simulink model "mcb_microchip_pmsm_foc_sensorless_dsPIC33EP256MC506"  (R2021b)
settings: Solver=FixedStepDiscrete  StartTime=0.0  StopTime=10  FixedStep=Ts  RelTol=1e-3  EnableMultiTasking=on
InitFcn:
  | mcb_microchip_pmsm_foc_sensorless_dsPIC33_data;
values from neighbouring files (symbols this model uses):
  dataType = fixdt(1,16,14)    [mcb_microchip_pmsm_foc_sensorless_dsPIC33_data.m]    (also in mcb_pmsm_foc_sensorless_dsPIC33_data.m)
  dataType2 = fixdt(1,16,12)    [mcb_microchip_pmsm_foc_sensorless_dsPIC33_data.m]    (also in mcb_pmsm_foc_sensorless_dsPIC33_data.m)
  PI_params = mcb.internal.SetControllerParameters(pmsm,inverter,PU_System,T_pwm,Ts,Ts_speed)    [mcb_microchip_pmsm_foc_sensorless_dsPIC33_data.m]    (also in mcb_pmsm_foc_sensorless_dsPIC33_data.m)
  PU_System = mcb_SetPUSystem(pmsm,inverter)    [mcb_microchip_pmsm_foc_sensorless_dsPIC33_data.m]    (also in mcb_pmsm_foc_sensorless_dsPIC33_data.m)
  PWM_frequency = 20e3    (= 20000)    [mcb_microchip_pmsm_foc_sensorless_dsPIC33_data.m]    (also in mcb_pmsm_foc_sensorless_dsPIC33_data.m)
  Speed_openLoop_PU = 0.1    [mcb_microchip_pmsm_foc_sensorless_dsPIC33_data.m]    (also in mcb_pmsm_foc_sensorless_dsPIC33_data.m)
  Ts = T_pwm    (= 5e-05)    [mcb_microchip_pmsm_foc_sensorless_dsPIC33_data.m]    (also in mcb_pmsm_foc_sensorless_dsPIC33_data.m)
  Ts_speed = 30*Ts    (= 0.0015)    [mcb_microchip_pmsm_foc_sensorless_dsPIC33_data.m]    (also in mcb_pmsm_foc_sensorless_dsPIC33_data.m)
undefined symbols (not defined in the file or in its folder): A4, C5, D8, F1, inverter, P20, P53, P97, Pin, pmsm, PWMmax
libraries: MCHP_Blockset x16, mcbcontrolslib x13, simulink x9, mcbpositiondecoderlib x2, mcbplantlib x1, autolibpmsmexterior x1
(part 1 of 3)
settings Model: Creator=M91449  LastModifiedBy=snarayan
settings SolverCC: AlgebraicLoopSolver=TrustRegion
settings DataIOCC: LimitDataPoints=on  ReturnWorkspaceOutputs=off
settings OptimizationCC: DefaultParameterBehavior=Inlined  InlineInvariantSignals=on  LifeSpan=1  EfficientTunableParamExpr=on
settings DebuggingCC: MultiTaskDSMMsg=none  SFUnexpectedBacktrackingDiag=warning  SFNoUnconditionalDefaultTransitionDiag=warning  SFExecutionAtInitializationDiag=none  SFMachineParentedDataDiag=warning  ArithmeticOperatorsInVariantConditions=warning
settings HardwareCC: ProdBitPerInt=16  ProdBitPerPointer=16  ProdBitPerSizeT=16  ProdBitPerPtrDiffT=16  ProdLargestAtomicInteger=Integer  ProdLargestAtomicFloat=None  ProdWordSize=16  ProdHWDeviceType=Generic->Custom
settings ModelReferenceCC: ModelReferenceNumInstancesAllowed=Single  PropagateSignalLabelsOutOfModel=off
settings SFSimCC: SimUseLocalCustomCode=off  MATLABDynamicMemAlloc=off  CustomCodeUndefinedFunction=UseInterfaceOnly
settings RTWCC: Description=Microchip Embedded Target PIC24 dsPIC30 dsPIC33 (real-time)  SystemTargetFile=MCHP_dsPIC_stf.tlc  TemplateMakefile=MCHP_dsPIC.tmf  GenerateReport=on  RTWUseLocalCustomCode=off  IncludeHyperlinkInReport=on  GenerateTraceInfo=on  GenerateTraceReport=on  GenerateTraceReportSl=on  GenerateTraceReportSf=on  GenerateTraceReportEml=on  GenerateCodeMetricsReport=on  GenerateCodeReplacementReport=on
settings CodeAppCC: IgnoreCustomStorageClasses=off  MaxIdLength=255  StateflowObjectComments=on
settings STFCustomTargetCC: TargetLibSuffix=_lib.a  CodeReplacementLibrary=Microchip Code Replacement Library for dsPIC  IncludeMdlTerminateFcn=off  CombineOutputUpdateFcns=on  SuppressErrorStatus=on  ERTCustomFileBanners=on  SupportContinuousTime=off  RemoveResetFunc=on  MATLABClassNameForMDSCustomization=Simulink.SoftwareTarget.ERTCustomization  GRTInterface=off  SystemTargetFile=MCHP_dsPIC_stf.tlc
settings ERTTargetCC: TargetLibSuffix=_lib.a  CodeReplacementLibrary=Microchip Code Replacement Library for dsPIC  MultiwordLength=2048  ParMdlRefBuildCompliant=off  CompOptLevelCompliant=off  ConcurrentExecutionCompliant=off  IncludeMdlTerminateFcn=off  SuppressErrorStatus=on  SupportNonInlinedSFcns=on  ModelStepFunctionPrototypeControlCompliant=off  CPPClassGenCompliant=off  UseToolchainInfoCompliant=off  InlinedParameterPlacement=NonHierarchical  ERTSrcFileBannerTemplate=MCHP_dsPIC_code_template.cgt  ERTHdrFileBannerTemplate=MCHP_dsPIC_code_template.cgt  ERTDataSrcFileTemplate=MCHP_dsPIC_code_template.cgt  ERTDataHdrFileTemplate=MCHP_dsPIC_code_template.cgt  ERTCustomFileTemplate=MCHP_main.tlc  ConvertIfToSwitch=off  SuppressUnreachableDefaultCases=off
settings ConfigComp: CovMetricSettings=dw  CovSaveCumulativeToWorkspaceVar=on  CovSaveSingleToWorkspaceVar=on  CovExternalEMLEnable=off

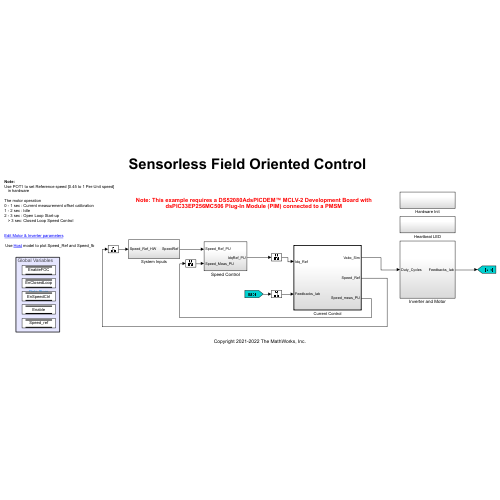
[thumbnail: Simulink's stored preview of the top-level diagram]
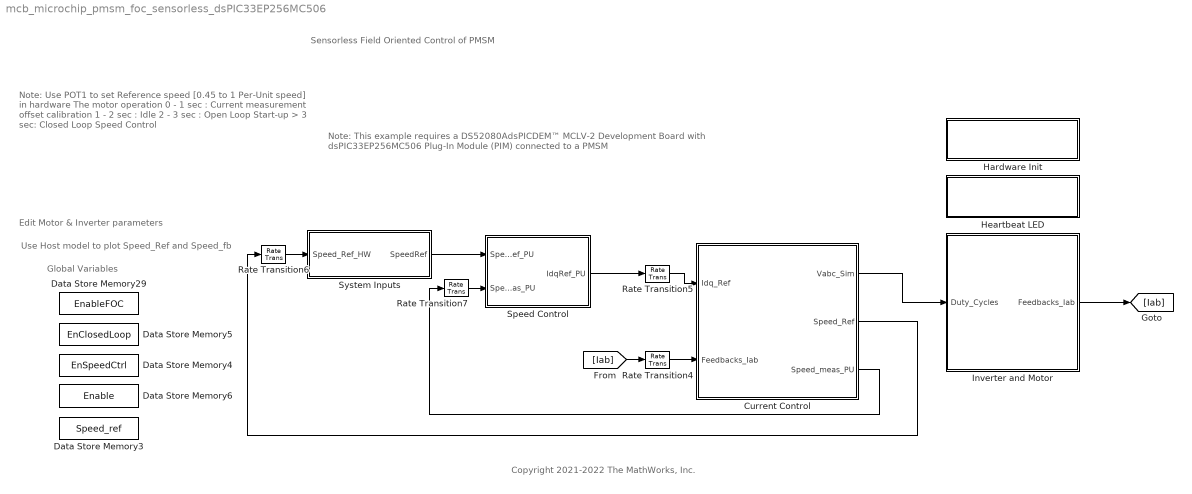
== system mcb_microchip_pmsm_foc_sensorless_dsPIC33EP256MC506 ==
  note: Use Host model to plot Speed_Ref and Speed_fb
  note: Edit Motor & Inverter parameters
  note: Note:
      | Use POT1 to set Reference speed [0.45 to 1 Per-Unit speed]
      | in hardware
      |
      | The motor operation
      | 0 - 1 sec : Current measurement offset calibration
      | 1 - 2 sec : Idle
      | 2 - 3 sec : Open Loop Start-up
      | > 3 sec: Closed Loop Speed Control
  note: Global Variables
  note: Sensorless Field Oriented Control of PMSM
  note: Note: This example requires a DS52080AdsPICDEM™ MCLV-2 Development Board with
      | dsPIC33EP256MC506 Plug-In Module (PIM) connected to a PMSM
  note: Copyright 2021-2022 The MathWorks, Inc.
  Current Control : Subsystem  TreatAsAtomicUnit=on  VariantControl=Optimized
  Data Store Memory29 : DataStoreMemory  DataStoreName=EnableFOC  ShowAdditionalParam=off  OutDataTypeStr=boolean
  Data Store Memory3 : DataStoreMemory  DataStoreName=Speed_ref  ReadBeforeWriteMsg=warning  WriteAfterWriteMsg=warning  WriteAfterReadMsg=warning  InitialValue=0.1  ShowAdditionalParam=off  OutDataTypeStr=dataType
  Data Store Memory4 : DataStoreMemory  DataStoreName=EnSpeedCtrl  ReadBeforeWriteMsg=warning  WriteAfterWriteMsg=warning  WriteAfterReadMsg=warning  ShowAdditionalParam=off  OutDataTypeStr=boolean
  Data Store Memory5 : DataStoreMemory  DataStoreName=EnClosedLoop  ReadBeforeWriteMsg=warning  WriteAfterWriteMsg=warning  WriteAfterReadMsg=warning  ShowAdditionalParam=off  OutDataTypeStr=boolean
  Data Store Memory6 : DataStoreMemory  DataStoreName=Enable  ShowAdditionalParam=off  OutDataTypeStr=boolean
  Hardware Init : Subsystem
  Heartbeat LED : Subsystem
  Inverter and Motor : Subsystem
  Rate Transition4 : RateTransition  Deterministic=off
  Rate Transition5 : RateTransition  Deterministic=off
  Rate Transition6 : RateTransition  Deterministic=off  OutPortSampleTime=Ts_speed
  Rate Transition7 : RateTransition  Deterministic=off  OutPortSampleTime=Ts_speed
  Speed Control : Subsystem  SystemSampleTime=Ts_speed
  System Inputs : Subsystem
  wires:
  Current Control/1(Vabc_Sim) -> Inverter and Motor/1(Duty_Cycles)
  Rate Transition4/1 -> Current Control/2(Feedbacks_Iab)
  Rate Transition7/1 -> Speed Control/2(Speed_Meas_PU)
  Speed Control/1(IdqRef_PU) -> Rate Transition5/1
  Current Control/3(Speed_meas_PU) -> Rate Transition7/1
  Inverter and Motor/1(Feedbacks_Iab) -> [Iab]
  [Iab] -> Rate Transition4/1
  Rate Transition5/1 -> Current Control/1(Idq_Ref)
  Current Control/2(Speed_Ref) -> Rate Transition6/1
  Rate Transition6/1 -> System Inputs/1(Speed_Ref_HW)
  System Inputs/1(SpeedRef) -> Speed Control/1(Speed_Ref_PU)

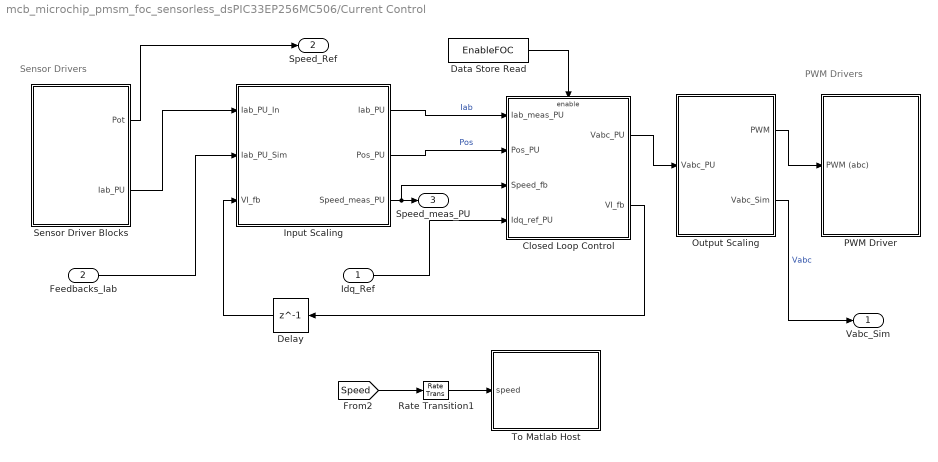
== system mcb_microchip_pmsm_foc_sensorless_dsPIC33EP256MC506/Current Control ==
  note: Sensor Drivers
  note: PWM Drivers
  Idq_Ref : Inport
  Feedbacks_Iab : Inport  Port=2
  Closed Loop Control : Subsystem
  Data Store Read : DataStoreRead  DataStoreName=EnableFOC  IndexOptions=Index vector (dialog)  Indices=1  OutputSizes=1
  Delay : Delay  DelayLength=1
  Input Scaling : Subsystem
  Output Scaling : Subsystem
  PWM Driver : Subsystem
  Rate Transition1 : RateTransition
  Sensor Driver Blocks : Subsystem
  "To Matlab Host " : Subsystem
  Vabc_Sim : Outport
  Speed_Ref : Outport  Port=2
  Speed_meas_PU : Outport  Port=3
  wires:
  Closed Loop Control/1(Vabc_PU) -> Output Scaling/1(Vabc_PU)
  Output Scaling/1(PWM) -> PWM Driver/1(PWM (abc))
  Feedbacks_Iab/1 -> Input Scaling/2(Iab_PU_Sim)
  Input Scaling/1(Iab_PU) -> Closed Loop Control/1(Iab_meas_PU)  "Iab"
  Input Scaling/2(Pos_PU) -> Closed Loop Control/2(Pos_PU)  "Pos"
  Sensor Driver Blocks/1(Pot) -> Speed_Ref/1
  Sensor Driver Blocks/2(Iab_PU) -> Input Scaling/1(Iab_PU_In)
  Rate Transition1/1 -> "To Matlab Host "/1(speed)
  [Speed] -> Rate Transition1/1
  Closed Loop Control/2(VI_fb) -> Delay/1
  Delay/1 -> Input Scaling/3(VI_fb)
  Idq_Ref/1 -> Closed Loop Control/4(Idq_ref_PU)
  Output Scaling/2(Vabc_Sim) -> Vabc_Sim/1  "Vabc"
  Input Scaling/3(Speed_meas_PU) -> Closed Loop Control/3(Speed_fb), Speed_meas_PU/1
  Data Store Read/1 -> Closed Loop Control/Enable

== system mcb_microchip_pmsm_foc_sensorless_dsPIC33EP256MC506/Hardware Init ==
  Compiler Options : MCHP_Blockset/System Configuration/Compiler Options  Priority=1  LATEST_CMPLR=on  COMP_LIST=Dynamic Options  COMP_LIST_TXT=xc16 - v1.70  DFP_LIST=Dynamic Options  DFP_LIST_TXT=Dynamic Options  CMSIS_DSP=Dynamic Options  CMSIS_DSP_TXT=Dynamic Options  USE_64BIT_DOUBLE=off  MCHP_MULTITHREAD_COMPILATION=on  UseCustom_LinkerScript=off  MCHP_MASTERLINK=mcb_pmsm_foc_sensorless_dsPIC33EP256MC506/Hardware Init/Microchip Master  OPTIMIZATION_LEVEL=3  OPTIMIZATION_FLTO=on  OPTIMIZATION_REORDER=off  UNROLL_LOOPS=on  PROCEDURAL_ABSTRACTION=off  MPLAB_LINKLIB=default  MPLAB_LINKLIB1=default  MCODE=is less than 32768 (faster)  MCONST=in data memory  MDATA=Use only memory below address 8192 (faster)  MSCALAR=Use only memory below address 8192 (faster)  MLARGEARRAY=off  MAGGREGATE=off  HEAP_SIZE=0  OMF=elf  DEBUG_INFO=off  ProduceHexOutput=on  AssemblyListing=off  NO_EDS_WARN=on  PRINT_STATISTICS=off
      settings: SourceProductName=MPLAB Device Blocks for Simulink
  Data Sheet : MCHP_Blockset/System Info/Data Sheet  DOC_Type=datasheet  DOC_MCHP_Id=33EP256MC506_datasheet  DOC_FilePath=C:\Users\M91449\AppData\Local\Temp\70000657H.pdf  DOC_FileLastCheckTime="[2016              1             28             13             25         44.133]"  cpy_MCHP_Id=33EP256MC506  MCHP_MASTERLINK=mcb_pmsm_foc_sensorless_dsPIC33EP256MC506/Hardware Init/Microchip Master
      settings: AttributesFormatString=%<cpy_MCHP_Id>  SourceProductName=MPLAB Device Blocks for Simulink
  Microchip Master : MCHP_Blockset/System Configuration/Microchip Master  Priority=1  PICREF=33EP256MC506  TIMESTEP_REF=ADC  BUSYFLAG=Dynamic Options  BUSYFLAG_TXT=D8 / Pin[42]  PWRTEN=Not used  BOREN=Disable  BODENV=2.7V  BORV=Not used  FPWRT=128ms  DSBOREN=Enable ZPBOR during Deep Sleep Mode  DSLPBOR=Not used  MCLRE=Enabled  SMCLR=MCLR pin generates a normal system Reset  PMDL1WAY=Allow only one reconfiguration  RSTPRI=Device will obtain reset instruction from Primary flash  TEMP=Not used  SOSCSRC=Not used  SOSCSEL=Not used  IOL1WAY=Allow only one reconfiguration  ALTVREF=Not used  DISUVREG=Not used  DSSWEN=Not used  LPCFG=Not used  RTCBAT=Not used  VBTBOR=Not used  WUTSEL=Not used  POWERSAVE=off  FNOSC=Primary Oscillator (XT; HS; EC)  FPR=ECIO w/ PLL 16x  FOSFPR=HS3 w/PLL 16x  FOS=Primary Oscillator  FRANGE=High Range  OSCILLATOR_SELECT=Crystal / Ceramic resonator  OSCILLATOR_SELECT_spd=Crystal / Ceramic resonator  QUARTZ=8e6  QUARTZ_spd=8e6  POSCGAIN=2x gain setting  POSCBOOST=Boost the kick start of the oscillator  SOSCGAIN=2x gain setting  SOSCBOOST=Boost the kick start of the oscillator  ACTIV_PLL=on  ACTIV_PLL_spd=on  MIPS_DESIRED=70e6  MIPS_DESIRED_spd=70e6  FPLLMUL=Not used  FPLLIDIV=8x Divider  POSCFREQ=Not used  POSCMD=XT Crystal Oscillator Mode  POSCMOD=Primary Oscillator Disabled  MIPS=70 * 1e6  ACLKCON=Optimized for PWM resolution & ADC conversion speed  ACLKCON_spd=Optimized for PWM resolution & ADC conversion speed  FPLLODIV=32x Divider  PLLKEN=Clock switch to PLL source will wait until the PLL lock signal is valid.  FCKSM=Both Clock switching and Fail-safe Clock Monitor are enabled  FCKSMEN=Sw Disabled; Mon Disabled  IESO=Start up with FRC; then switch  DSWDTPS=1:2^36  FWDTEN=Disable  FWDTWINSZ=Window size is 25%  FWPSA=1:512  FWPSA0=1:128  FWPSB=1:16  WDT=Disable  WDTPOST=1:32768  WDTPRE=1:128  WDTPS=1:32768  WINDIS=Watchdog Timer in Non-Window mode  WWDTEN=Non-Window mode  DSWDTEN=Enable DSWDT during Deep Sleep Mode  DSWDTOSC=Select LPRC as DSWDT Reference clock  FPBDIV=Not used  FSOSCEN=Disable Secondary Oscillator  LPRCSEL=Not used  OSCIOFCN=Not used  OSCIOFNC=general purpose digital I/O pin  LVRCFG=Not used  PLL_96MHZ=Not used  PLL96MHZ=Not used  PLLDIV=Not used  WDTCLK=Not used  WDTCMX=Not used  WDTWIN=WDT Window is 25% of WDT period  XTCFG=24-32 MHz crystals  XTBST=Boost the kick-start  APL=Aux Flash Code protect is disabled  APLK=Aux Flash Write Protection or Code Protection is Enabled  AWRP=Auxiliary program memory is not write-protected  BSS=No Boot program Flash segment  BWP=Not used  BWRP=Boot Segment may be written  CP=Protection Disabled  EBS=No Boot EEPROM  ESS=No Segment Data EEPROM  GCP=General Segment Code protect is Disabled  GSS=General Segment Code protect is Disabled  GSS0=Not used  GSSK=General Segment Write Protection or Code Protection is Enabled  GWRP=General Segment may be written  PWP=Not used  RBS=No Boot RAM  RSS=No Secure RAM  SSS=No Secure Segment  SWRP=Secure segment may be written  WPCFG=Not used  WPDIS=Not used  WPEND=Not used  WPFP=Not used  ICESEL=Communicate on PGEC1/PGED1  ICS=Communicate on PGEC2 and PGED2  JTAGEN=Disable  COE=Not used  RES=Not used  DEBUG=Debugger is disabled  BACKBUG=Not used  BKBUG=Not used  ALTI2C=I2C mapped to SDA1/SCL1 pins  ALTI2C1=I2C1 mapped to SDA1/SCL1 pins  ALTI2C2=I2C2 mapped to SDA2/SCL2 pins  ALTI2C3=I2C3 mapped to SDA3/SCL3 pins  ALTQIO=QEA1; QEB1; INDX1 are selected as inputs to QEI1  ALTSS1=SS1A is selected as the I/O pin for SPI1  CMPPOL0=Hysteresis is applied to falling edge  CMPPOL1=Hysteresis is applied to falling edge  FCANIO=Not used  FETHIO=Default Ethernet I/O  FMIIEN=MII Enabled  FSRSSEL=Not used  FUSBIDIO=Controlled by the USB Module  FVBUSONIO=Not used  HPOL=PWM module high side output pins have active-high output polarity  HYST0=45 mV Hysteresis  HYST1=45 mV Hysteresis  I2C1SEL=Not used  LPOL=PWM module low side output pins have active-high output polarity  PWMPIN=PWM module pins controlled by PORT register at device Reset  RTCOSC=Not used  UPLLEN=USB PLL Disabled  UPLLIDIV=Not used  ATMOD8=Not used  ALTPMP=Not used  I2C2SEL=Not used  ALTADREF=Not used  ALTCVREF=Not used  PWMLOCK=PWM registers may be written without key sequence  INT_PRIORITY_DMA=0  MCHP_TIMER_RESULT=[ ]  MCHP_PORT={Busy Flag}{Busy}0:1:D8;  MCHP_PLLRegisters="[5    243  16385     -1     -1]"  MCHPVAR=MCHP.fcy.MIPS=70000000;MCHP.fcy.SYSCLK=70000000;MCHP.fcy.ADC=70000000;MCHP.fcy.Comparator=70000000;MCHP.fcy.I2C=70000000;MCHP.fcy.SPI=70000000;MCHP.fcy.UART=70000000;MCHP.fcy.Timers=70000000;MCHP.fcy.OC=70000000;MCHP.fcy.IC=70000000;MCHP.fcy.Ports=70000000;MCHP.fcy.QEI=70000000;MCHP.PowerSave=0;MCHP.TimeStepFactor=-1000;MCHP.TimeStep_Timer=-1;MCHP.NTIMERS=5;MCHP.id.name='33EP256MC506';MCHP.id.N=reshape([33 256 506],1,3);MCHP.id.L=reshape({ 'EP','MC',''},1,3);MCHP.id.Arch=3;MCHP.periph.PPS.reg_RPINRx=reshape([-1 1 1 -1 -1 -1 1 -1 -1 -1 -1 -1 -1 -1 1 1 1 1 -1 -1 -1 -1 -1 -1 1 1 -1 -1 1 1 1 1 -1 -1 -1 -1 1 -1 1 -1 -1 -1 -1 -1 1 1 1 -1 -1 -1 -1 -1 1 -1 -1 -1 -1 -1 -1 -1 -1 -1 -1 -1 -1 -1 -1 -1 -1 -1 -1 -1 -1 -1 -1 1 -1 1 1 1],1,80);MCHP.PPS.dsPIC.RP=reshape([-1 -1 -1 -1 -1 -1 -1 -1 -1 -1 -1 -1 -1 -1 -1 -1 -1 -1 -1 -1 4 -1 -1 -1 -1 -1 -1 -1 -1 -1 -1 -1 -1 -1 -1 19 20 21 22 23 24 25 26 27 -1 -1 -1 -1 -1 -1 -1 -1 -1 -1 38 39 40 41 -1 -1 -1 -1 -1 -1 -1 -1 -1 -1 -1 -1 -1 -1 -1 -1 -1 -1 -1 -1 -1 -1 -1 -1 -1 -1 -1 -1 -1 -1 -1 -1 -1 -1 -1 -1 -1 -1 -1 81 -1 -1 -1 -1 -1 -1 -1 -1 -1 -1 -1 -1 -1 -1 -1 -1 -1 -1 -1 -1 102 -1 104],1,121);MCHP.PPS.dsPIC.RPI=reshape([-1 -1 -1 -1 -1 -1 -1 -1 -1 -1 -1 -1 -1 -1 -1 -1 -1 -1 -1 -1 -1 -1 -1 -1 8 9 -1 11 12 -1 -1 -1 16 17 18 -1 -1 -1 -1 -1 -1 -1 -1 -1 28 29 30 31 -1 -1 -1 35 36 37 -1 -1 -1 -1 42 -1 -1 -1 -1 -1 -1 -1 -1 -1 -1 -1 -1 -1 -1 -1 -1 -1 -1 -1 -1 -1 -1 -1 -1 -1 -1 -1 -1 -1 -1 -1 -1 -1 -1 -1 78 79 80 -1 -1 -1 -1 -1 -1 -1 -1 -1 -1 -1 -1 -1 -1 -1 -1 -1 -1 -1 -1 -1 -1 103 -1 105],1,122);MCHP.PPS.dsPIC.RPINR_list=reshape({ '1','INT1','INT2','INT3','INT4','T1CK','T2CK','T3CK','T4CK','T5CK','T6CK','T7CK','T8CK','T9CK','IC1','IC2','IC3','IC4','IC5','IC6','IC7','IC8','OCFA','OCFB','FLT1','FLT2','FLT3','FLT4','QEIA1','QEIB1','QEINDX1','QEIHOM1','QEIA2','QEIB2','QEINDX2','QEIHOM2','U1RX','U1CTS','U2RX','U2CTS','SDI1','SCK1_in','SS1_in','44','SDI2','SCK2_in','SS2_in','48','CSDIR','CSCK','COFS','52','C1RX','C2RX','U3RX','U3CTS','U4RX','U4CTS','SDI3','SCK3_in','SS3_in','62','SDI4','SCK4_in','SS4_in','66','IC9','IC10','IC11','IC12','IC13','IC14','IC15','IC16','OCFC','SYNCI1','SYNCI2','DTCMP1','DTCMP2','DTCMP3','DTCMP4','DTCMP5','DTCMP6','DTCMP7','FLT5','FLT6','FLT7','FLT8','89','SENT1','SENT2','92'},1,92);MCHP.PPS.dsPIC.RPOR_list=reshape({ '1','U1TX','U1RTS','U2TX','U2RTS','SDO1','SCK1_out','SS1_out','SDO2','SCK2_out','SS2_out','CSDO','CSCK','COFS','C1TX','C2TX','OC1','OC2','OC3','OC4','OC5','OC6','OC7','OC8','C1OUT','C2OUT','C3OUT','U3TX','U3RTS','U4TX','U4RTS','SDO3','SCK3_out','SS3_out','SDO4','SCK4_out','SS4_out','OC9','OC10','OC11','OC12','OC13','OC14','OC15','OC16','SYNCO1','SYNCO2','QEI1CCMP','QEI2CCMP','REFCLK','C4OUT','C5OUT','52','53','54','55','56','SENT1','SENT2'},1,59);MCHP.PPS.map_RPnR_RPORx=reshape([20 35 36 37 38 39 40 41 42 43 54 55 56 57 -1 97 -1 118 120],1,19);MCHP.Rx=reshape([13 15 21 -1 -1 58 -1 -1 -1 -1 -1 14 16 22 -1 -1 59 -1 -1 -1 -1 -1 -1 17 23 -1 -1 -1 -1 -1 -1 -1 -1 -1 18 35 -1 -1 -1 -1 -1 -1 -1 -1 33 32 36 -1 -1 -1 -1 -1 -1 -1 -1 -1 43 37 53 -1 -1 -1 -1 -1 -1 -1 -1 44 50 54 -1 -1 4 -1 -1 -1 -1 1 46 51 -1 -1 -1 5 -1 -1 -1 -1 31 48 52 42 -1 -1 6 -1 -1 -1 -1 34 49 55 -1 -1 -1 8 -1 -1 -1 -1 64 60 45 -1 -1 -1 -1 -1 -1 -1 -1 12 61 24 -1 -1 -1 -1 -1 -1 -1 -1 11 62 39 -1 27 -1 -1 -1 -1 -1 -1 -1 63 47 -1 28 -1 -1 -1 -1 -1 -1 -1 2 -1 -1 29 -1 -1 -1 -1 -1 -1 -1 3 40 -1 30 -1 -1 -1 -1 -1 -1],11,16);MCHP.ADC.ANtype=reshape([3 0],1,2);MCHP.ADC.ADCONx=reshape([47103 59391 40959 263 0 0],1,6);MCHP.ADC.ADCHS_0=reshape([40863 1799],1,2);MCHP.ADC.Flags=reshape([1 0],1,2);MCHP.ADC.Buffer=reshape([16 -1],1,2);MCHP.ADC.port=reshape([0 1 16 17 18 19 32 33 34 11 12 43 76 77 78 79 -1 -1 -1 -1 -1 -1 -1 -1 -1 -1 -1 -1 -1 -1 -1 -1 -1 -1 -1 -1 -1 -1 -1 -1 -1 -1 -1 -1 -1 -1 -1 -1 -1 -1 -1 -1 -1 -1 -1 -1 -1],1,57);MCHP.ADC.port_ALT=reshape([-1 -1 -1 -1],1,4);MCHP.ADC.port_VrefP=17;MCHP.ADC.port_VrefM=16;MCHP.ADC.port_AVdd=-1;MCHP.ADC.port_AVss=-1;MCHP.ADC.ADCDATA=reshape([0 0 0 0 0 0 0 0 0 0 0 0 0 0 0 0 0 0 0 0 0 0 0 0 0 0 0 0 0 0 0 0 0 0 0 0 0 0 0 0 0 0 0 0 0 0 0 0 0 0 0 0 0 0 0 0 0],1,57);MCHP.ADC.HS_SAR.TRGSRC=reshape([0 0 0 0 0 0 0 0 0 0 0 0 0 0 0 0 0 0 0 0 0 0 0 0 0 0],1,26);MCHP.ADC.HS_SAR.nFilters=0;MCHP.ADC.HS_SAR.nDedicatedCore=0;MCHP.ADC.HS_SAR.CALIBRATION=0;MCHP.ADC.HS_SAR.ADCON1L=-1;MCHP.ADC.HS_SAR.ADC_Class3_idxStart=32;MCHP.memory.RAM=32768;MCHP.memory.RAM_XBegin=4096;MCHP.memory.RAM_YBegin=20480;MCHP.memory.RAM_dma=reshape([-1 -1],1,2);MCHP.memory.FLASH_ECC=0;MCHP.DMA.Num=4;MCHP.DMA.CNTmax=16383;MCHP.QEI.QEICONx=reshape([49023 -1 -1 -1 -1 -1],1,6);MCHP.QEI.QEItype=1;MCHP.QEI.Port_QEI_INDX=reshape([-1 -1],1,2);MCHP.QEI.Port_QEI_QEA=reshape([-1 -1],1,2);MCHP.QEI.Port_QEI_QEB=reshape([-1 -1],1,2);MCHP.QEI.Port_QEI_UPDN=reshape([-1 -1],1,2);MCHP.INT.Port=reshape([23 32767 32767 -1 -1],1,5);MCHP.PWM_HS.Flags=reshape([3 1 0],1,3);MCHP.PWM.port_FLT=reshape([-1 -1 -1 34 43 -1 -1 -1 -1 -1 -1 -1 -1 -1 -1 -1 -1 -1 -1 -1 -1 -1 -1 -1 -1 -1 -1 -1 -1 -1 -1 -1 20],1,33);MCHP.PWM.PWMRef=-1;MCHP.PWM.Flag=0;MCHP.PWM.Port_PWM_l=reshape([31 -1 29 -1 27 -1 -1 -1 -1 -1 -1 -1 -1 -1 -1 -1 -1 -1 -1 -1 -1 -1 -1 -1],2,12);MCHP.PWM.Port_PWM_h=reshape([30 -1 28 -1 26 -1 -1 -1 -1 -1 -1 -1 -1 -1 -1 -1 -1 -1 -1 -1 -1 -1 -1 -1],2,12);MCHP.PWM_HS_FEP.nEVTOUT=-1;MCHP.IC.Port=reshape([32767 32767 32767 32767 0 0 0 0 0 0 0 0 0 0 0 0],1,16);MCHP.IC.type=1;MCHP.OC.Port=reshape([32767 32767 32767 32767 0 0 0 0 0 0 0 0 0 0 0 0],1,16);MCHP.OC.type=1;MCHP.CN.Port=reshape([-1 -1 -1 -1 -1 -1 -1 -1 -1 -1 -1 -1 -1 -1 -1 -1 -1 -1 -1 -1 -1 -1 -1 -1 -1 -1 -1 -1 -1 -1 -1 -1 -1 -1 -1 -1 -1 -1 -1 -1 -1 -1 -1 -1 -1 -1 -1 -1 -1 -1 -1 -1 -1 -1 -1 -1 -1 -1 -1 -1 -1 -1 -1 -1 -1 -1 -1 -1 -1 -1 -1 -1 -1 -1 -1 -1 -1 -1 -1 -1 -1 -1 -1 -1 -1],1,85);MCHP.CN.PullUp=reshape([8083 65535 49151 352 61440 3 960 0 0 0 0],1,11);MCHP.CN.type=1;MCHP.CN.Flag_PullDown=1;MCHP.SPI.Refs=reshape([1 2 0 0 0 0],1,6);MCHP.SPI.SPIxCON1=8191;MCHP.SPI.SPIxCON2=57347;MCHP.SPI.Port_SDI=reshape([9 -1 -1 -1 -1 -1],1,6);MCHP.SPI.Port_SDO=reshape([4 -1 -1 -1 -1 -1],1,6);MCHP.SPI.Port_SCK=reshape([35 -1 -1 -1 -1 -1],1,6);MCHP.SPI.Port_SS=reshape([16 -1 -1 -1 -1 -1],1,6);MCHP.I2C.Refs=reshape([1 2 0 0 0],1,5);MCHP.I2C.I2CxCON=49151;MCHP.I2C.NewRegName=1;MCHP.I2C.Port_SDA=reshape([36 8 -1 -1 -1],1,5);MCHP.I2C.Port_SCL=reshape([37 20 -1 -1 -1],1,5);MCHP.I2C.Port_ASDA=reshape([25 21 -1 -1 -1],1,5);MCHP.I2C.Port_ASCL=reshape([24 22 -1 -1 -1],1,5);MCHP.I2C.Fuse_Port_SCL_SDA=reshape([3 1 4 1 -1 -1 -1 -1 -1 -1],2,5);MCHP.I2C.Fuse_Port_ASCL_ASDA=reshape([3 2 4 2 -1 -1 -1 -1 -1 -1],2,5);MCHP.SCCP.nSCCP=0;MCHP.SCCP.MCCP=reshape([0 0 0 0 0 0 0 0 0],1,9);MCHP.PGA.Port_PGA1P=reshape([-1 -1 -1 -1],1,4);MCHP.PGA.Port_PGA1N=reshape([-1 -1 -1 -1],1,4);MCHP.PGA.Port_PGA2P=reshape([-1 -1 -1 -1],1,4);MCHP.PGA.Port_PGA2N=reshape([-1 -1 -1 -1],1,4);MCHP.PGA.Num=0;MCHP.HS_AnalogComparator.Port_CMP1=reshape([-1 -1 -1 -1],1,4);MCHP.HS_AnalogComparator.Port_CMP2=reshape([-1 -1 -1 -1],1,4);MCHP.HS_AnalogComparator.Port_CMP3=reshape([-1 -1 -1 -1],1,4);MCHP.HS_AnalogComparator.Port_CMP4=reshape([-1 -1 -1 -1],1,4);MCHP.HS_AnalogComparator.PORT_EXTREFx=reshape([-1 -1],1,2);MCHP.HS_AnalogComparator.Port_DACOUTx=reshape([-1 -1],1,2);MCHP.HS_AnalogComparator.Num=0;MCHP.Comp.Port_CVrefin=-1;MCHP.Comp.Port_CVref=-1;MCHP.Comp.Port_CVref1O=24;MCHP.Comp.Port_CVref2O=4;MCHP.Comp.Port_CxOUT=reshape([32767 32767 32767 32767 -1],1,5);MCHP.Comp.Port_OAxOUT=reshape([17 0 32 -1 -1],1,5);MCHP.Comp.Port_CxINP=reshape([18 1 34 32 -1],1,5);MCHP.Comp.Port_CxINM=reshape([19 43 -1 -1 16 76 -1 -1 33 77 -1 -1 33 -1 -1 -1 -1 -1 -1 -1],4,5);MCHP.Comp.Port_OAxINP=reshape([-1 -1 -1 -1 -1],1,5);MCHP.Comp.Port_OAxINM=reshape([-1 -1 -1 -1 -1],1,5);MCHP.Comp.nComp=reshape([4 0 0],1,3);MCHP.Comp.OpAmp=7;MCHP.Comp.CVRCON=reshape([17663 0],1,2);MCHP.Comp.CMCON=0;MCHP.CDAC.Port_DACx=reshape([-1 -1 -1],1,3);MCHP.CDAC.nCDAC=0;MCHP.UART.port_Rx=reshape([32767 32767 -1 -1 -1 -1],1,6);MCHP.UART.port_Tx=reshape([32767 32767 -1 -1 -1 -1],1,6);MCHP.UART.port_ARx=reshape([-1 -1],1,2);MCHP.UART.port_ATx=reshape([-1 -1],1,2);MCHP.UART.port_RTS=reshape([34 76 -1 -1 -1 -1],1,6);MCHP.UART.port_CTS=reshape([43 77 -1 -1 -1 -1],1,6);MCHP.UART.reg_UxMODE=reshape([48127 48127 -1 -1 -1 -1],1,6);MCHP.UART.reg_UxSTA=reshape([61439 61439 -1 -1 -1 -1],1,6);MCHP.modsrc.DOS_02551_cpu_16bit_v7=0;MCHP.modsrc.DOS_01520_wdt_dmt_upb_v1_16bit=0;MCHP.modsrc.DOS_02359a_sent_j2716_upb_v1=0;MCHP.modsrc.DOS_02672_math_progcrc_upb_v1_16bit=0;MCHP.modsrc.DOS_01577_cla_clc_upb_v1=0;MCHP.modsrc.DOS_02915_ecc_v2=0;MCHP.modsrc.DOS_02673_tmr_classa_upb_v1_16bit=0;MCHP.modsrc.DOS_01494_qei_32b_upb_v1_16bit=0;MCHP.modsrc.DOS_02552_msi_upb_v1_Master=0;MCHP.modsrc.DOS_01441_i2c_upb_v1_16bit_TLAH=0;MCHP.modsrc.DOS_03076_uart_protocol_upb_v1_16bit=0;MCHP.modsrc.DOS_01482=0;MCHP.modsrc.DOS_01483_pwm_16bit=0;MCHP.modsrc.DOS_02497_WACV=0;MCHP.modsrc.DOS_02316_nvm_ctrl_v1_16bit=0;MCHP.modsrc.DOS_02653_afe_current_bias_ctrl_upb_v1_16bit=0;MCHP.modsrc.DOS_01459_ptg_pc_upb_v1_16bit=0;MCHP.modsrc.DOS_01512_ccp_mccp_upb_v1_16bit=0;MCHP.modsrc.DOS_02519_dma_sfr_16bit_v2=0;MCHP.modsrc.DOS_02508c11=0;MCHP.modsrc.DOS_02475_dac_pdm_nbit_upb_v1_16bit=0;MCHP.modsrc.DOS_02467_gpio_upb_v1_16bit=0;MCHP.modsrc.DOS_00805_rst_integration_v4=0;MCHP.modsrc.DOS_02659_clk_sib_v12=0;MCHP.modsrc.DOS_02674_wdt_upb_v1_16bit=0;MCHP.modsrc.DOS_01407=0;MCHP.modsrc.DOS_02552_msi_upb_v1_Slave=0;MCHP.modsrc.DOS_02593_amp_pga_ctrl_pb_v2_16bit=0;MCHP.modsrc.DOS_03247_CAN_FD_UPB_V2_16_bit=0;MCHP.modsrc.DOS_01461_afe_ctmu_con_upb_v1_16bit=0;MCHP.modsrc.DOS_02497_WACA=0;MCHP.modsrc.DOS_02478_uart_irda_upb_v1_16bit=0;MCHP.modsrc.DOS_00929=1;MCHP.modsrc.DOS_01198=1;MCHP.modsrc.DOS_03029_WACH=0;MCHP.modsrc.DOS_02949_WACG=0;MCHP.modsrc.DOS_03349_amp_pad_opamp_ctrl_upb_v1=0;MCHP.modsrc.DOS_02237_osc_dco_ctrl_upb_v1_16bit=0;MCHP.modsrc.DOS_02472_ppi_pmp16_upb_v1_16bit=0;MCHP.modsrc.DOS_03994_WAC07=0;MCHP.modsrc.DOS_03662_WACU=0;MCHP.modsrc.DOS_00794=1;MCHP.modsrc.DOS_00931=1;MCHP.modsrc.DOS_00932=1;MCHP.modsrc.DOS_00942=1;MCHP.modsrc.DOS_00938=1;MCHP.modsrc.DOS_00996=1;MCHP.modsrc.DOS_00997=1;MCHP.modsrc.DOS_00998=1;MCHP.modsrc.DOS_00209=0;MCHP.modsrc.DOS_01555_adc=0;MCHP.modsrc.DOS_01293=1;MCHP.modsrc.DOS_00828=0;MCHP.modsrc.DOS_01116=1;MCHP.modsrc.DOS_01017_RPORx=1;MCHP.modsrc.DOS_01017_RPINRx=1;MCHP.modsrc.DOS_01555_nvm_tsmc18_v2_16bit=0;MCHP.modsrc.DOS_00804=1;MCHP.modsrc.DOS_00826=1;MCHP.modsrc.DOS_01555_TLAK_PMDx=0;MCHP.modsrc.DOS_01555_TLAK_INT_=0;MCHP.modsrc.DOS_00933=1;MCHP.modsrc.DOS_01555=0;MCHP.modsrc.DOS_01555_ptg=0;MCHP.modsrc.DOS_00958=1;MCHP.modsrc.DOS_01117_PORTx=1;MCHP.modsrc.DOS_00999=0;MCHP.modsrc.DOS_01041=1;MCHP.modsrc.DOS_00892=1;MCHP.modsrc.DOS_01287_TLAC_PMDx=1;MCHP.modsrc.DOS_01287_TLAC_INT_=1;MCHP.modsrc.DOS_01424=1;MCHP.modsrc.DOS_01332=1;MCHP.modsrc.DOS_01468_PMBA_current_source=0;MCHP.modsrc.DOS_02291_PGA=0;MCHP.modsrc.DOS_01467_Comparator=0;MCHP.modsrc.DOS_01498_TLAY=0;MCHP.modsrc.DOS_00993_PLL_120MHz=0;MCHP.modsrc.DOS_01332_ptg_pc_v1=0;MCHP.modsrc.DOS_00958_pwm_TLAY=0;MCHP.modsrc.TLAY_IOPorts=0;MCHP.modsrc.DOS_00929q=0;MCHP.modsrc.DOS_02415_spi_v5=0;MCHP.modsrc.DOS_RPINRx_16bit_2=0;MCHP.modsrc.DOS_01497_TLAH_PMDx=0;MCHP.modsrc.DOS_02550_TLAL_INT=0;MCHP.modsrc.DOS_00958_pwm_TLAH=0;MCHP.modsrc.DOS_01287_TLAH_INT_=0;MCHP.modsrc.DOS_01113=0;MCHP.modsrc.DOS_01017_PMDx=0;MCHP.modsrc.DOS_00927=0;MCHP.modsrc.DOS_01080=0;MCHP.modsrc.DOS_00794_cpu_16bit_v3=0;MCHP.modsrc.DOS_02192_TLCD_PMDx=0;MCHP.modsrc.DOS_02192_TLCD_INT_=0;MCHP.modsrc.DOS_02192_cmp=0;MCHP.modsrc.DOS_00958_pwm_TLCD=0;MCHP.modsrc.DOS_02192_PORTx_TLCD=0;MCHP.modsrc.DOS_00936=0;MCHP.modsrc.DOS_00995=0;MCHP.modsrc.DOS_00546=0;MCHP.modsrc.DOS_00474=0;MCHP.modsrc.DOS_02481_WACK_MC_Config=0;MCHP.modsrc.DOS_03088_pfm_cache_ocp_v2_WACK=0;MCHP.modsrc.DOS_02819_pfm_ctrl_32bit_upb_v2=0;MCHP.modsrc.DOS_02674_wdt_upb_v1_32bit=0;MCHP.modsrc.DOS_01520_wdt_dmt_upb_v1=0;MCHP.modsrc.DOS_02869_icd_jtag_bvci_upb_v2=0;MCHP.modsrc.DOS_02823_WACJ_clk_cru_upb_v2=0;MCHP.modsrc.DOS_02823_WACN_clk_cru_upb_v2=0;MCHP.modsrc.DOS_01423_RPINRx=0;MCHP.modsrc.DOS_02481_RPORx=0;MCHP.modsrc.DOS_02511_pwr_sib_upb_v1_32bit=0;MCHP.modsrc.DOS_02907_WACN_GP_int_evic_v3=0;MCHP.modsrc.DOS_01500_dma_bvci_v2=0;MCHP.modsrc.DOS_02141_tmr_classa_pb_v2=0;MCHP.modsrc.DOS_02815_tmr_classb_upb_v1=0;MCHP.modsrc.DOS_00740_icap_pb_v1=0;MCHP.modsrc.DOS_00749_ocmp_pb_v1=0;MCHP.modsrc.DOS_01441_i2c_upb_v1_32bit=0;MCHP.modsrc.DOS_01329_spi_pb_v2=0;MCHP.modsrc.DOS_02478_uart_irda_upb_v1_32bit=0;MCHP.modsrc.DOS_03554_cmp_control_upb_v2_32bit=0;MCHP.modsrc.DOS_01445_dac_nbit__control_upb_v1_32bit=0;MCHP.modsrc.DOS_01461_afe_ctmu_con_upb_v1=0;MCHP.modsrc.DOS_01577_cla_clc_upb_v1_32bit=0;MCHP.modsrc.DOS_02467_gpio_ports_upb_v1=0;MCHP.modsrc.DOS_02508_adc_sar_ctrl_upb_v1_PIC32MK=0;MCHP.modsrc.DOS_01261_tmr_rtcc_pb_v2=0;MCHP.modsrc.DOS_01475_lpwr_deep_sleep_ctrl_v2=0;MCHP.modsrc.DOS_EIP_00136_ssx_v1=0;MCHP.modsrc.DOS_02907_WACN_MC_int_evic_v3=0;MCHP.modsrc.DOS_01477_pwm_mc_upb_v1=0;MCHP.modsrc.DOS_01494_qei_32b_upb_v1=0;MCHP.modsrc.DOS_03247_can_fd_upb_v2_pic32mk=0;MCHP.modsrc.DOS_02907_WACK_MC_int_evic_v3=0;MCHP.modsrc.DOS_02514_dfm_strl_sst_upb_v1=0;MCHP.modsrc.DOS_02472_ppi_pmp16_upb_v1=0;MCHP.modsrc.DOS_02813a_usb_otgcore_pb_v3=0;MCHP.modsrc.DOS_02481_WACJ_MC_Config=0;MCHP.modsrc.DOS_02569_pfm_cache_ocp_v1=0;MCHP.modsrc.DOS_02481_WACJ_MC_int_evic_v3=0;MCHP.modsrc.DOS_01459_ptg_pc_upb_v1_SIC=0;MCHP.modsrc.DOS_01427_cmp_control_upb_v1_32bit=0;MCHP.modsrc.DOS_01152_can_bvci_v1=0;MCHP.modsrc.DOS_02787_WACD_Config=0;MCHP.modsrc.DOS_00800_dac_4bit_ctrl_pb_v1=0;MCHP.modsrc.DOS_01539_icd_jtag_pb_v2=0;MCHP.modsrc.DOS_02823_clk_cru_upb_v2=0;MCHP.modsrc.DOS_01423_RPORx=0;MCHP.modsrc.DOS_02907_WACD_int_evic_v3=0;MCHP.modsrc.DOS_00734_uart_irda_pb_v1=0;MCHP.modsrc.DOS_00687_tmr_classa_pb_v1=0;MCHP.modsrc.DOS_00745_tmr_classb_pb_v1=0;MCHP.modsrc.DOS_02508_adc_sar_ctrl_upb_v1=0;MCHP.modsrc.DOS_00866_cmp_control_pb_v2=0;MCHP.modsrc.DOS_01114_eth_bvci_v1=0;MCHP.modsrc.DOS_02831_usb_clk_rst_v2=0;MCHP.modsrc.DOS_01643_pfm_cache_ahb_v2=0;MCHP.modsrc.DOS_EIP_00206r5_sqi_v2=0;MCHP.modsrc.DOS_EIP_00124_usb_hs_otgcore_v1=0;MCHP.modsrc.DOS_EIP_00218_math_rng_ahbs_v2=0;MCHP.modsrc.DOS_EIP_00109_ebi_v1=0;MCHP.modsrc.DOS_EIP_00158_crypto_v1=0;MCHP.PortBase=16;MCHP.PortPrefixe='P';MCHP.clock.PBxDIV=-1;  MCHP_CRC=15317496  BTMODE=Not used  RES1=Not used  PLLSS=Not used  RES2=Not used  ALTCMPI=Not used  BOREN1=Not used  ALTRB6=Not used  RETCFG=Not used  DFMCY=Not used  BSS2=No Boot Segment  BSEN=No Boot Segment  CWRP=Configuration Segment may be written  CSS=No Protection (other than CWRP)  AIVTDIS=Disable Alternate Vector Table  BSLIM=Not used  WDTEN=Disable  BTSWP=BOOTSWP instruction is disabled  DBCC=No Cross Connection between DAC outputs  CTXT1=Not Assigned  CTXT2=Not Assigned  SEQNUM=Not used  nSEQNUM=Not used  BOREN0=Enabled  DMTIVT=Not used  DMTCNT=2^31 (2147483648)  DMTEN=Dead Man Timer is Disabled and can be enabled by software  ON=Not used  USERID=Not used  RESERVED1=Not used  PGL1WAY=Allow only one reconfiguration  FPLLRNG=34-68 MHz Input  FPLLICLK=FRC is input to the System PLL  FPLLMULT=PLL Multiply by 128  UPLLFSEL=USB PLL input is 24 MHz  DMTINTV=Window/Interval value is 127/128 counter value  WDTSPGM=WDT stops during Flash programming  FDMTEN=Deadman Timer is disabled  TRCEN=Trace features in the CPU are enabled  BOOTISA=Boot code and Exception code is MIPS32  FECCCON=ECC and Dynamic ECC are disabled (ECCCON bits are writable)  EXTDDRSIZE=Not used  FSLEEP=Flash is powered down when the device is in Sleep mode  DBGPER=Allow CPU access to all permission regions  EJTAGBEN=Normal EJTAG functionality  TSEQ=Not used  CSEQ=Not used  RWDTPS=1:1048576  RCLKSEL=Always use LPRC  SWDTPS=1:1048576  DMTIVTL=Not used  DMTIVTH=Not used  DMTCNTL=Not used  DMTCNTH=Not used  DMTDIS=Dead Man Timer is Disabled and can be enabled by software  SMBEN=SMBus input threshold is enabled  SPI2PIN=SPI2 uses I/O remap (PPS) pins  CTXT3=Not Assigned  CTXT4=Not Assigned  MBXM0=Mailbox register configured for Master data read (Slave to Master data transfer)  MBXM1=Mailbox register configured for Master data read (Slave to Master data transfer)  MBXM2=Mailbox register configured for Master data read (Slave to Master data transfer)  MBXM3=Mailbox register configured for Master data read (Slave to Master data transfer)  MBXM4=Mailbox register configured for Master data read (Slave to Master data transfer)  MBXM5=Mailbox register configured for Master data read (Slave to Master data transfer)  MBXM6=Mailbox register configured for Master data read (Slave to Master data transfer)  MBXM7=Mailbox register configured for Master data read (Slave to Master data transfer)  MBXM8=Mailbox register configured for Master data read (Slave to Master data transfer)  MBXM9=Mailbox register configured for Master data read (Slave to Master data transfer)  MBXM10=Mailbox register configured for Master data read (Slave to Master data transfer)  MBXM11=Mailbox register configured for Master data read (Slave to Master data transfer)  MBXM12=Mailbox register configured for Master data read (Slave to Master data transfer)  MBXM13=Mailbox register configured for Master data read (Slave to Master data transfer)  MBXM14=Mailbox register configured for Master data read (Slave to Master data transfer)  MBXM15=Mailbox register configured for Master data read (Slave to Master data transfer)  MBXHSA=MSIxMBXD15 assigned to mailbox handshake protocol block A  MBXHSB=MSIxMBXD15 assigned to mailbox handshake protocol block B  MBXHSC=MSIxMBXD15 assigned to mailbox handshake protocol block C  MBXHSD=MSIxMBXD15 assigned to mailbox handshake protocol block D  MBXHSE=MSIxMBXD15 assigned to mailbox handshake protocol block E  MBXHSF=MSIxMBXD15 assigned to mailbox handshake protocol block F  MBXHSG=MSIxMBXD15 assigned to mailbox handshake protocol block G  MBXHSH=MSIxMBXD15 assigned to mailbox handshake protocol block H  HSAEN=Mailbox data flow control handshake protocol block disabled.  HSBEN=Mailbox data flow control handshake protocol block disabled.  HSCEN=Mailbox data flow control handshake protocol block disabled.  HSDEN=Mailbox data flow control handshake protocol block disabled.  HSEEN=Mailbox data flow control handshake protocol block disabled.  HSFEN=Mailbox data flow control handshake protocol block disabled.  HSGEN=Mailbox data flow control handshake protocol block disabled.  HSHEN=Mailbox data flow control handshake protocol block disabled.  CPRA0=Master core owns pin.  CPRA1=Master core owns pin.  CPRA2=Master core owns pin.  CPRA3=Master core owns pin.  CPRA4=Master core owns pin.  CPRB0=Master core owns pin.  CPRB1=Master core owns pin.  CPRB2=Master core owns pin.  CPRB3=Master core owns pin.  CPRB4=Master core owns pin.  CPRB5=Master core owns pin.  CPRB6=Master core owns pin.  CPRB7=Master core owns pin.  CPRB8=Master core owns pin.  CPRB9=Master core owns pin.  CPRB10=Master core owns pin.  CPRB11=Master core owns pin.  CPRB12=Master core owns pin.  CPRB13=Master core owns pin.  CPRB14=Master core owns pin.  CPRB15=Master core owns pin.  CPRC0=Master core owns pin.  CPRC1=Master core owns pin.  CPRC2=Master core owns pin.  CPRC3=Master core owns pin.  CPRC4=Master core owns pin.  CPRC5=Master core owns pin.  CPRC6=Master core owns pin.  CPRC7=Master core owns pin.  CPRC8=Master core owns pin.  CPRC9=Master core owns pin.  CPRC10=Master core owns pin.  CPRC11=Master core owns pin.  CPRC12=Master core owns pin.  CPRC13=Master core owns pin.  CPRC14=Master core owns pin.  CPRC15=Master core owns pin.  CPRD0=Master core owns pin.  CPRD1=Master core owns pin.  CPRD2=Master core owns pin.  CPRD3=Master core owns pin.  CPRD4=Master core owns pin.  CPRD5=Master core owns pin.  CPRD6=Master core owns pin.  CPRD7=Master core owns pin.  CPRD8=Master core owns pin.  CPRD9=Master core owns pin.  CPRD10=Master core owns pin.  CPRD11=Master core owns pin.  CPRD12=Master core owns pin.  CPRD13=Master core owns pin.  CPRD14=Master core owns pin.  CPRD15=Master core owns pin.  CPRE0=Master core owns pin.  CPRE1=Master core owns pin.  CPRE2=Master core owns pin.  CPRE3=Master core owns pin.  CPRE4=Master core owns pin.  CPRE5=Master core owns pin.  CPRE6=Master core owns pin.  CPRE7=Master core owns pin.  CPRE8=Master core owns pin.  CPRE9=Master core owns pin.  CPRE10=Master core owns pin.  CPRE11=Master core owns pin.  CPRE12=Master core owns pin.  CPRE13=Master core owns pin.  CPRE14=Master core owns pin.  CPRE15=Master core owns pin.  S1FNOSC=Internal Fast RC (FRC) Oscillator with postscaler  S1IESO=Start up with FRC; then switch  S1OSCIOFNC=OSC2 is clock output  S1FCKSM=Both Clock switching and Fail-safe Clock Monitor are disabled  S1PLLKEN=S1PLLKEN_ON  S1RWDTPS=1:1048576  S1RCLKSEL=Always use LPRC  S1WINDIS=Watchdog Timer operates in Non-Window mode  S1WDTWIN=WDT Window is 25% of WDT period  S1SWDTPS=1:1048576  S1FWDTEN=Disable  S1ICS=Communicate on PGC1 and PGD1  S1DEBUG=Not used  S1ISOLAT=The slave can operate (in debug mode) even if the SLVEN bit in the MSI is zero.  S1NOBTSWP=BOOTSWP instruction is disabled  S1ALTI2C1=I2C1 mapped to SDA1/SCL1 pins  S1SPI1PIN=Slave SPI1 uses I/O remap (PPS) pins  S1SSRE=Slave generated resets will reset the Slave Enable Bit in the MSI module  S1MSRE=The master software oriented RESET events (RESET Op-Code; Watchdog timeout; TRAP reset; illegalInstruction) will also cause the slave subsystem to reset.  S1CTXT1=Not Assigned  S1CTXT2=Not Assigned  S1CTXT3=Not Assigned  S1CTXT4=Not Assigned  BORLVL=Not used  BSSO=Not used  MCA=Not used  MAXTEMP=Not used  CFGAN14=Not used  CFGAN15=Not used  S1IOL1WAY=Not used  S1BSSO=Not used  S1BACKBUG=Not used  BISTDIS=mBIST on reset feature disabled  NOBTSWP=BOOTSWP instruction is disabled  S1BISTDIS=Slave BIST on reset feature disabled  S1DMTIVTL=Not used  S1DMTIVTH=Not used  S1DMTCNTL=Not used  S1DMTCNTH=Not used  S1DMTDIS=Slave Dead Man Timer is Disabled and can be enabled by software  BSEQ=Not used  IBSEQ=Not used  SMB3EN=SMBus 3.0 input levels  FUSBIDIO2=USBID pin is controlled by the USB2 module  FVBUSIO2=VBUSON pin is controlled by the USB2 module  FUSBIDIO1=USBID pin is controlled by the USB1 module  FVBUSIO1=VBUSON pin is controlled by the USB1 module  VBATBOREN=Enable ZPBOR during VBAT Mode  FDSEN=Enable DSEN bit in DSCON  BORSEL=BOR trip voltage 2.1v (Non-OPAMP deviced operation)  POSCFGAIN=Gain is G3  POSCAGCDLY=Settling time = 25ms x AGCRNG  POSCAGCRNG=Range 1x  POSCAGC=Automatic Gain Control for Oscillator  FDBGWP=Not used
      settings: SourceProductName=MPLAB Device Blocks for Simulink
  Model Info : simulink/Model-Wide Utilities/Model Info  Frame=on  DisplayStringWithTags=|  HorizontalTextAlignment=Left  LeftAlignmentValue=0.02
      | Long hust motor with:
      | M1 - Black
      | M2 - Red
      | M3 - White
      | 
      | Encoder on HA - HB 
      | HA: Blue wire
      | HB: White wire
  Open Board and Motor pages : Subsystem
      settings: OpenFcn=|
      | web('www.microchip.com/DevelopmentTools/ProductDetails.aspx?PartNO=DM330021-2','-browser');
      | pause(1);
      | web('http://www.microchipdirect.com/productsearch.aspx?keywords=AC300020','-browser');
      | pause(1);
      | web('www.microchipdirect.com/ProductSearch.aspx?keywords=AC300022','-browser');
      mask Display: disp('Open tools\nWebpage');
  Port Info : MCHP_Blockset/System Info/Port Info  MCHP_MASTERLINK=mcb_pmsm_foc_sensorless_dsPIC33EP256MC506/Hardware Init/Microchip Master
      settings: SourceProductName=MPLAB Device Blocks for Simulink
  Tasks State Show base rate Task on pin D8 (PIM) : MCHP_Blockset/Profiling/Tasks State  TasksPin=D8  MCHP_PORT={Task D1 Running}{Task D1}15:1:D8;  MCHP_MASTERLINK=mcb_pmsm_foc_sensorless_dsPIC33EP256MC506/Hardware Init/Microchip Master
      settings: SourceProductName=MPLAB Device Blocks for Simulink
  Timer Info : MCHP_Blockset/System Info/Timer Info  MCHP_MASTERLINK=mcb_pmsm_foc_sensorless_dsPIC33EP256MC506/Hardware Init/Microchip Master
      settings: SourceProductName=MPLAB Device Blocks for Simulink
  UART Configuration : MCHP_Blockset/BUS UART/UART Configuration  UART_REF=2  BAUD_Choice=Dynamic Options  BAUD_Choice_TXT="3000000         [-2.78%]"  BAUD_Choice_IR=Dynamic Options  BAUD_Choice_IR_TXT=[]  BAUD_Custom=115200  INT_PRIORITY=0  ALT_IO=on  PIN_RX=Dynamic Options  PIN_RX_TXT=C5 / P53 / Pin[37]  PIN_TX=Dynamic Options  PIN_TX_TXT=F1 / P97 / Pin[59]  MCHP_PORT="{UART2  Tx}{U2TX}3:1:P97;"  MCHP_MASTERLINK=mcb_pmsm_foc_sensorless_dsPIC33EP256MC506/Hardware Init/Microchip Master  MCHP_COM_ExtPil=off  TX_IMPLEMENTATION=Circular Buffer  TX_IMPLEMENTATION_default=Circular Buffer  TX_INT_PRIORITY=5  TX_INT_WHEN=is empty & last char is sent  TX_INT_WHEN_default=is empty & last char is sent  TX_CIRCULAR_SIZE=64  TX_DMA_CHANNEL="0   (Lowest Priority)"  TX_DMA_SIZE=60  TX_TASK_PROTECTION=Delay tasks (default)  TX_INTERRUPT_PROTECTION=Do not send on conflict (default)  TX_INTERRUPT_PROTECTION_default=Do not send on conflict (default)  RX_IMPLEMENTATION=Do not implement Rx  RX_IMPLEMENTATION_default=Circular Buffer  RX_INT_PRIORITY=1  RX_INT_WHEN=receive 1 character  RX_CIRCULAR_SIZE=32  RX_DMA_CHANNEL=0  RX_DMA_SIZE=0  DuplexMode=Full duplex (default)  PIN_RX_Inv=off  PIN_TX_Inv=off  PIN_RXTX_Inv=off  ParityBit=No parity (default)  StopBit=1 stop bit (default)  IRDA=off  FlowControl=None  PIN_CTS=Dynamic Options  PIN_CTS_TXT=A4 / P20 / Pin[33]  PIN_RTS=Dynamic Options  PIN_RTS_TXT=A4 / P20 / Pin[33]  InitSequence_chkbox=off  BAUD_Choice_InitSeq=Dynamic Options  BAUD_Choice_InitSeq_TXT="110         [-0.00%]"  BAUD_Choice_IR_InitSeq=Dynamic Options  BAUD_Choice_IR_InitSeq_TXT=0  BAUD_Custom_InitSeq=0  InitSequence='Hello World'
      settings: SourceProductName=MPLAB Device Blocks for Simulink

== system mcb_microchip_pmsm_foc_sensorless_dsPIC33EP256MC506/Heartbeat LED ==
  Counter Free-Running : simulink/Sources/Counter Free-Running  NumBits=1  tsamp=0.5
  Data Type Conversion : DataTypeConversion  OutDataTypeStr=boolean
  LED 1 : MCHP_Blockset/Digital IO/Digital Output  PORT=Dynamic Options  PORT_TXT="D   [ 5  6  8 ]"  PIN=6  PACK=off  SIMULTANEOUS=off  READPREVIOUS=off  ORDERING=None  SampleTime=-1  MCHP_MASTERLINK=mcb_pmsm_foc_sensorless_dsPIC33EP256MC506/Hardware Init/Microchip Master
      settings: SourceProductName=MPLAB Device Blocks for Simulink
  wires:
  Data Type Conversion/1 -> LED 1/1
  Counter Free-Running/1 -> Data Type Conversion/1

== system mcb_microchip_pmsm_foc_sensorless_dsPIC33EP256MC506/Inverter and Motor ==
  Duty_Cycles : Inport
  Codegeneration : Subsystem
  Simulation : Subsystem
  Variant Sink : VariantSink
  Variant Source : VariantSource
  Feedbacks_Iab : Outport  VectorParamsAs1DForOutWhenUnconnected=off
  wires:
  Codegeneration/1(Feedbacks_Iab) -> Variant Source/1
  Variant Sink/1 -> Codegeneration/1(Duty_Cycles)
  Simulation/1(Feedbacks_Iab) -> Variant Source/2
  Variant Sink/2 -> Simulation/1(Duty_Cycles)
  Variant Source/1 -> Feedbacks_Iab/1
  Duty_Cycles/1 -> Variant Sink/1

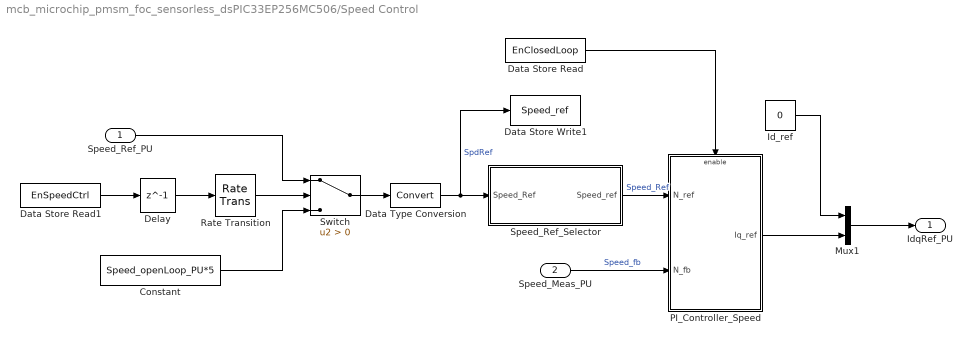
== system mcb_microchip_pmsm_foc_sensorless_dsPIC33EP256MC506/Speed Control ==
  Speed_Ref_PU : Inport
  Speed_Meas_PU : Inport  Port=2
  Constant : Constant  Value=Speed_openLoop_PU*5  OutDataTypeStr=Inherit: Inherit via back propagation
  Data Store Read : DataStoreRead  DataStoreName=EnClosedLoop  IndexOptions=Index vector (dialog)  Indices=1  OutputSizes=1
  Data Store Read1 : DataStoreRead  DataStoreName=EnSpeedCtrl  SampleTime=Ts_speed * 100  IndexOptions=Index vector (dialog)  Indices=1  OutputSizes=1
  Data Store Write1 : DataStoreWrite  DataStoreName=Speed_ref  IndexOptions=Index vector (dialog)  Indices=1  OutputSizes=1
  Data Type Conversion : DataTypeConversion
  Delay : Delay  DelayLength=1  UseCircularBuffer=on
  Id_ref : Constant  Value=0  OutDataTypeStr=dataType  SampleTime=Ts_speed
  Mux1 : Mux  Inputs=2
  PI_Controller_Speed : Subsystem
  Rate Transition : RateTransition  Integrity=off  Deterministic=off
  Speed_Ref_Selector : Subsystem
  Switch : Switch  Criteria=u2 > Threshold
  IdqRef_PU : Outport  VectorParamsAs1DForOutWhenUnconnected=off
  wires:
  Speed_Meas_PU/1 -> PI_Controller_Speed/2(N_fb)  "Speed_fb"
  Id_ref/1 -> Mux1/1
  Mux1/1 -> IdqRef_PU/1
  Data Store Read/1 -> PI_Controller_Speed/Enable
  PI_Controller_Speed/1(Iq_ref) -> Mux1/2
  Data Store Read1/1 -> Delay/1
  Rate Transition/1 -> Switch/2
  Data Type Conversion/1 -> Speed_Ref_Selector/1(Speed_Ref), Data Store Write1/1  "SpdRef"
  Switch/1 -> Data Type Conversion/1
  Constant/1 -> Switch/3
  Speed_Ref_PU/1 -> Switch/1
  Delay/1 -> Rate Transition/1
  Speed_Ref_Selector/1(Speed_ref) -> PI_Controller_Speed/1(N_ref)  "Speed_Ref"

== system mcb_microchip_pmsm_foc_sensorless_dsPIC33EP256MC506/System Inputs ==
  note: Note: Valid speed input is 0.3 to 0.75.
  Speed_Ref_HW : Inport
  Adjust Pot output : Subsystem
  Sim : Subsystem
  Variant Source1 : VariantSource
  SpeedRef : Outport
  wires:
  Variant Source1/1 -> SpeedRef/1
  Speed_Ref_HW/1 -> Adjust Pot output/1(In1)
  Adjust Pot output/1(Out1) -> Variant Source1/1
  Sim/1(Out1) -> Variant Source1/2

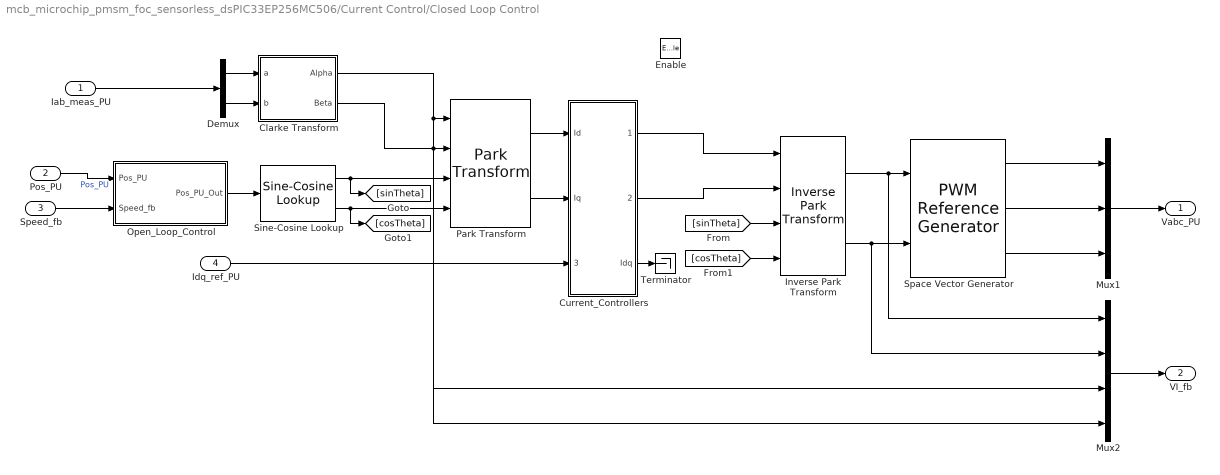
== system mcb_microchip_pmsm_foc_sensorless_dsPIC33EP256MC506/Current Control/Closed Loop Control ==
  Iab_meas_PU : Inport
  Pos_PU : Inport  Port=2
  Speed_fb : Inport  Port=3
  Idq_ref_PU : Inport  Port=4
  Enable : EnablePort
  Clarke Transform : Subsystem  AncestorBlock=mcbcontrolslib/Clarke Transform  TreatAsAtomicUnit=on  VariantControl=Variant2  mask(Clarke Transform){}
      mask help:
      | <p>Compute Clarke transformation on balanced 3-phase inputs into balanced 2-phase orthogonal outputs.
      | <br>
      | <br>
      | The block accepts two signals out of three phases, and outputs corresponding &alpha;-&beta; axis components, where phase-a axis is aligned with alpha axis.</p>
      mask Help: eval('mcb.internal.helpview(''clarketransform'')')
      mask Display: mcb.internal.drawIcons('Clarke',1);
  Current_Controllers : Subsystem
  Demux : Demux  Outputs=2
  Inverse Park Transform : mcbcontrolslib/Inverse Park Transform  AxisAlignment=D-axis
  Mux1 : Mux  Inputs=3
  Mux2 : Mux
  Open_Loop_Control : Subsystem
  Park Transform : mcbcontrolslib/Park Transform  AxisAlignment=D-axis
      settings: SourceProductBaseCode=MT
  Sine-Cosine Lookup : mcbcontrolslib/Sine-Cosine Lookup  AngleInput=Per-unit  N_points=1024
      settings: SourceProductBaseCode=MT
  Space Vector Generator : mcbcontrolslib/PWM Reference Generator  inSignal=Valphabeta  modType=SVM: space vector modulation
      settings: SourceProductBaseCode=MT
  Terminator : Terminator
  Vabc_PU : Outport  OutputWhenDisabled=reset  InitialOutput=[0 0 0]  VectorParamsAs1DForOutWhenUnconnected=off
  VI_fb : Outport  Port=2  OutputWhenDisabled=reset  InitialOutput=[0 0 0 0]  VectorParamsAs1DForOutWhenUnconnected=off
  wires:
  Current_Controllers/1(Vd_ref) -> Inverse Park Transform/1
  [sinTheta] -> Inverse Park Transform/3
  Sine-Cosine Lookup/1 -> [sinTheta], Park Transform/3
  Space Vector Generator/1 -> Mux1/1
  Space Vector Generator/3 -> Mux1/3
  Sine-Cosine Lookup/2 -> Park Transform/4, [cosTheta]
  Space Vector Generator/2 -> Mux1/2
  Idq_ref_PU/1 -> Current_Controllers/3(Idq_ref_PU)
  Iab_meas_PU/1 -> Demux/1
  Demux/1 -> Clarke Transform/1(a)
  Demux/2 -> Clarke Transform/2(b)
  Park Transform/2 -> Current_Controllers/2(Iq)
  [cosTheta] -> Inverse Park Transform/4
  Current_Controllers/2(Vq_ref) -> Inverse Park Transform/2
  Mux1/1 -> Vabc_PU/1
  Speed_fb/1 -> Open_Loop_Control/2(Speed_fb)
  Current_Controllers/3(Idq) -> Terminator/1
  Park Transform/1 -> Current_Controllers/1(Id)
  Pos_PU/1 -> Open_Loop_Control/1(Pos_PU)  "Pos_PU"
  Open_Loop_Control/1(Pos_PU_Out) -> Sine-Cosine Lookup/1
  Mux2/1 -> VI_fb/1
  Inverse Park Transform/1 -> Mux2/1, Space Vector Generator/1
  Clarke Transform/2(Beta) -> Mux2/4, Park Transform/2
  Inverse Park Transform/2 -> Space Vector Generator/2, Mux2/2
  Clarke Transform/1(Alpha) -> Mux2/3, Park Transform/1

== system mcb_microchip_pmsm_foc_sensorless_dsPIC33EP256MC506/Current Control/Input Scaling ==
  Iab_PU_In : Inport
  Iab_PU_Sim : Inport  Port=2
  VI_fb : Inport  Port=3
  DC component removal : Subsystem
  Sensorless : Subsystem
  Variant Source : VariantSource
  Iab_PU : Outport
  Pos_PU : Outport  Port=2
  Speed_meas_PU : Outport  Port=3
  tag scope: Speed=global
  wires:
  Iab_PU_Sim/1 -> Variant Source/2
  Variant Source/1 -> Iab_PU/1
  DC component removal/1(SigOUT) -> Sensorless/1(VI_fb)
  VI_fb/1 -> DC component removal/1(SigIN)  "Pos"
  Sensorless/2(Theta) -> Pos_PU/1  "Pos"
  Sensorless/1(Speed_meas_PU) -> [Speed], Speed_meas_PU/1
  Iab_PU_In/1 -> Variant Source/1

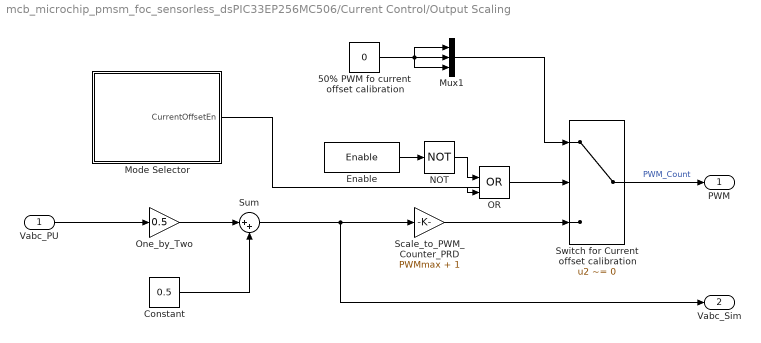
== system mcb_microchip_pmsm_foc_sensorless_dsPIC33EP256MC506/Current Control/Output Scaling ==
  Vabc_PU : Inport
  50% PWM fo current offset calibration : Constant  Value=0  OutDataTypeStr=Inherit: Inherit via back propagation
  Constant : Constant  Value=0.5  OutDataTypeStr=dataType  SampleTime=-1
  Enable : DataStoreRead  DataStoreName=Enable  IndexOptions=Index vector (dialog)  Indices=1  OutputSizes=1
  Mode Selector : Subsystem
  Mux1 : Mux  Inputs=3
  NOT : Logic  Operator=NOT  IconShape=distinctive  AllPortsSameDT=off  OutDataTypeStr=boolean
  OR : Logic  Operator=OR  IconShape=distinctive  AllPortsSameDT=off  OutDataTypeStr=boolean
  One_by_Two : Gain  Gain=0.5  RndMeth=Simplest  OutDataTypeStr=Inherit: Same as input
  Scale_to_PWM_Counter_PRD : Gain  Gain=PWMmax + 1  OutDataTypeStr=uint16  RndMeth=Simplest
  Sum : Sum  Inputs=|++
  Switch for Current offset calibration : Switch  Criteria=u2 ~= 0  Threshold=250
  PWM : Outport
  Vabc_Sim : Outport  Port=2
  wires:
  Constant/1 -> Sum/2
  One_by_Two/1 -> Sum/1
  Vabc_PU/1 -> One_by_Two/1
  Mux1/1 -> Switch for Current offset calibration/1
  50% PWM fo current offset calibration/1 -> Mux1/1, Mux1/3, Mux1/2
  Mode Selector/1(CurrentOffsetEn) -> OR/2
  OR/1 -> Switch for Current offset calibration/2
  Enable/1 -> NOT/1
  NOT/1 -> OR/1
  Scale_to_PWM_Counter_PRD/1 -> Switch for Current offset calibration/3
  Sum/1 -> Vabc_Sim/1, Scale_to_PWM_Counter_PRD/1
  Switch for Current offset calibration/1 -> PWM/1  "PWM_Count"
